simulink model "simple"  (Simulink 4.00)
settings: Solver=ode45  StartTime=0.0  StopTime=10.0  RelTol=1e-3
libraries: simulink3 x1, truetime x1
settings Model: Creator=anton  LastModifiedBy=anton  ExtModeAutoUpdateStatusClock=off

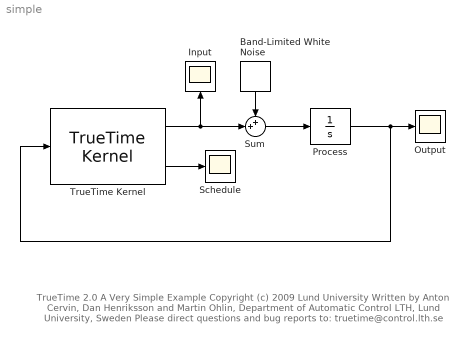
== system simple ==
  note: TrueTime 2.0  A Very Simple Example
      | Copyright (c) 2009 Lund University
      | Written by Anton Cervin, Dan Henriksson and Martin Ohlin,
      | Department of Automatic Control LTH, Lund University, Sweden
      | Please direct questions and bug reports to: truetime@control.lth.se
  Band-Limited White Noise : simulink3/Sources/Band-Limited White Noise  Orientation=down  Cov=[0.1]  Ts=0.1  seed=[23341]
  Input : Scope
      settings: Orientation=up  TimeRange=10  YMin=-1  YMax=1  SaveToWorkspace=off  SaveName=ScopeData2  LimitDataPoints=on  MaxDataPoints=5000
  Output : Scope
      settings: TimeRange=10  YMin=-1  YMax=1  SaveToWorkspace=off  LimitDataPoints=on  MaxDataPoints=5000
  Process : Integrator  ExternalReset=none  InitialConditionSource=internal  InitialCondition=0  LimitOutput=off  UpperSaturationLimit=inf  LowerSaturationLimit=-inf  ShowSaturationPort=off  ShowStatePort=off  AbsoluteTolerance=auto
  Schedule : Scope
      settings: TimeRange=auto  YMin=0  YMax=2  SaveToWorkspace=off  SaveName=ScopeData  MaxDataPoints=5000
  Sum : Sum  Inputs=++|  SaturateOnIntegerOverflow=on
  TrueTime Kernel : truetime/TrueTime Kernel  sfun=simple_init  args=[]  ninputsoutputs=[1 1]  ntriggers=0  trigtype=falling  nwnodenbr=[]  clockoffsetdrift=[0 0]  schedoutput=on  battery=off  poweroutput=off
  wires:
  TrueTime Kernel/2 -> Schedule/1
  TrueTime Kernel/1 -> Input/1, Sum/2
  Process/1 -> Output/1, TrueTime Kernel/1
  Sum/1 -> Process/1
  Band-Limited White Noise/1 -> Sum/1
